simulink model "moto_control"  (R2026a)
settings: Solver=VariableStepAuto  StopTime=3.0
settings Model: Creator=Charu  LastModifiedBy=Charu

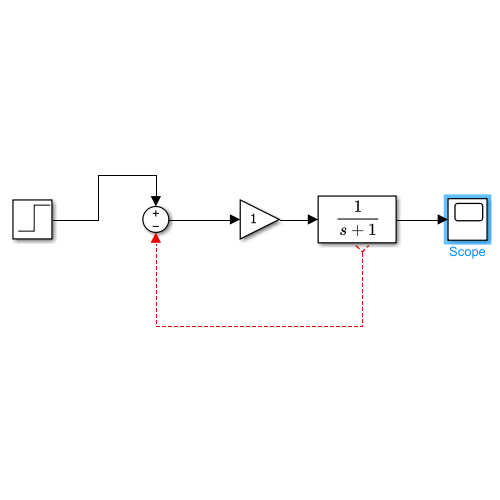
[thumbnail: Simulink's stored preview of the top-level diagram]
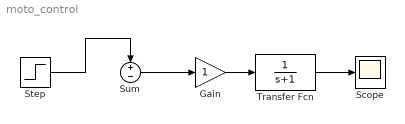
== system moto_control ==
  Gain : Gain
  Scope : Scope
      settings: ActiveDisplayYMinimum=-1.7125240519847464  ActiveDisplayYMaximum=5.2726358895982344
  Step : Step  SampleTime=0
  Sum : Sum  Inputs=+-
  Transfer Fcn : TransferFcn  Denominator=[1 1]
  wires:
  Gain/1 -> Transfer Fcn/1
  Transfer Fcn/1 -> Scope/1
  Sum/1 -> Gain/1
  Step/1 -> Sum/1
  ? -> Sum/2
